simulink model "SubSystemFuerPDRegler2"  (R2017a)
settings: Solver=VariableStepAuto  StartTime=0.0  StopTime=10.0  RelTol=1e-3
undefined symbols (not defined in the file or in its folder): Kd, Ks, T, T1, Td, Ts
settings Model: Creator=Christian  LastModifiedBy=prt01

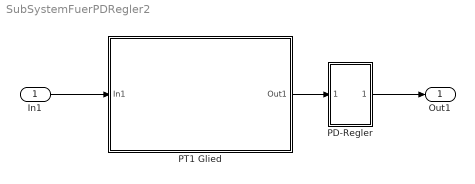
== system SubSystemFuerPDRegler2 ==
  In1 : Inport
  "PD-Regler " : Subsystem
  "PT1 Glied " : Subsystem
  Out1 : Outport
  wires:
  "PD-Regler "/1(Out1) -> Out1/1
  In1/1 -> "PT1 Glied "/1(In1)
  "PT1 Glied "/1(Out1) -> "PD-Regler "/1(In1)

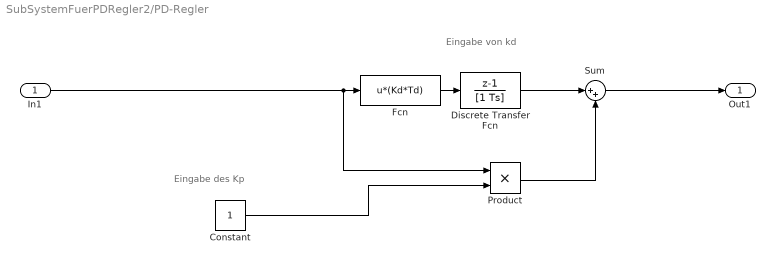
== system SubSystemFuerPDRegler2/PD-Regler  ==
  note: Eingabe von kd
  note: Eingabe des Kp
  In1 : Inport
  Constant : Constant
  Discrete Transfer Fcn : DiscreteTransferFcn  Numerator=[1 -1]  Denominator=[1 Ts]
  Fcn : Fcn  Expr=u*(Kd*Td)
  Product : Product
  Sum : Sum  Inputs=|++
  Out1 : Outport
  wires:
  Sum/1 -> Out1/1
  Product/1 -> Sum/2
  Constant/1 -> Product/2
  In1/1 -> Fcn/1, Product/1
  Discrete Transfer Fcn/1 -> Sum/1
  Fcn/1 -> Discrete Transfer Fcn/1

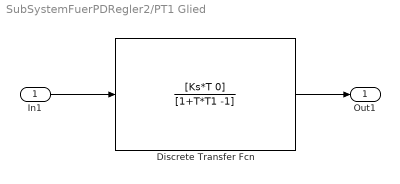
== system SubSystemFuerPDRegler2/PT1 Glied  ==
  In1 : Inport
  Discrete Transfer Fcn : DiscreteTransferFcn  Numerator=[Ks*T 0]  Denominator=[1+T*T1 -1]
  Out1 : Outport
  wires:
  Discrete Transfer Fcn/1 -> Out1/1
  In1/1 -> Discrete Transfer Fcn/1
